simulink model "MIT2"  (R2018a)
settings: Solver=VariableStepAuto  StartTime=0.0  StopTime=200  RelTol=1e-3
settings Model: Creator=boomboom  LastModifiedBy=edward
settings CodeAppCC: StateflowObjectComments=on

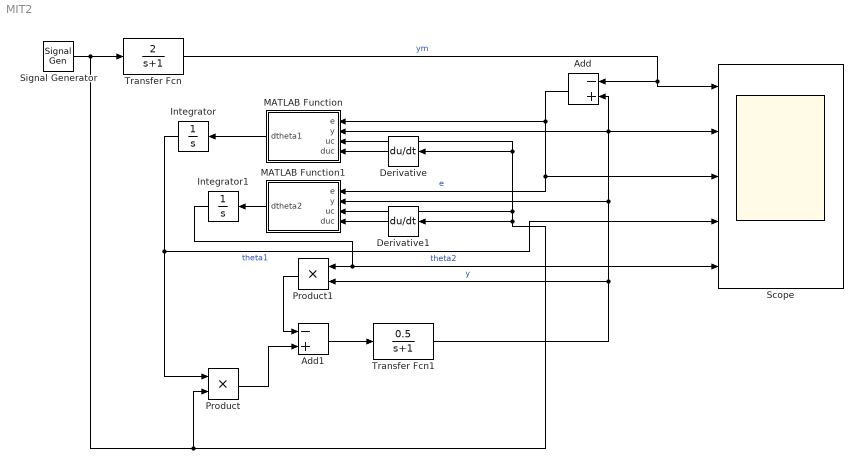
== system MIT2 ==
  Add : Sum  Inputs=-+
  Add1 : Sum  Inputs=-+
  Derivative : Derivative
  Derivative1 : Derivative
  Integrator : Integrator
  Integrator1 : Integrator
  MATLAB Function : MATLAB Function  TreatAsAtomicUnit=on
  MATLAB Function1 : MATLAB Function  TreatAsAtomicUnit=on
  Product : Product
  Product1 : Product
  Scope : Scope  NumInputPorts=5
  Signal Generator : SignalGenerator  Frequency=0.1  Units=rad/sec
  Transfer Fcn : TransferFcn  Numerator=[2]  Denominator=[1 1]
  Transfer Fcn1 : TransferFcn  Numerator=[0.5]  Denominator=[1 1]
  wires:
  Signal Generator/1 -> Product/2, Derivative1/1, Derivative/1, MATLAB Function/3(uc), MATLAB Function1/3(uc), Transfer Fcn/1
  Transfer Fcn/1 -> Add/1, Scope/1  "ym"
  Product/1 -> Add1/2
  Add1/1 -> Transfer Fcn1/1
  Product1/1 -> Add1/1
  Transfer Fcn1/1 -> Product1/2, MATLAB Function1/2(y), MATLAB Function/2(y), Add/2, Scope/2  "y"
  Add/1 -> Scope/3, MATLAB Function1/1(e), MATLAB Function/1(e)  "e"
  Derivative/1 -> MATLAB Function/4(duc)
  Derivative1/1 -> MATLAB Function1/4(duc)
  MATLAB Function/1(dtheta1) -> Integrator/1
  Integrator/1 -> Scope/4, Product/1  "theta1"
  MATLAB Function1/1(dtheta2) -> Integrator1/1
  Integrator1/1 -> Scope/5, Product1/1  "theta2"

== matlab function MIT2/MATLAB Function1 ==
  data: e input; dtheta2 output; y input; uc input; duc input
function dtheta2 = fcn(e,y,uc,duc)
am=2;
bm=2;
a=1;
b=0.5;
gamma=0.2
dtheta2 = -gamma*(am/(duc+am*y))*e

== matlab function MIT2/MATLAB Function ==
  data: e input; dtheta1 output; y input; uc input; duc input
function dtheta1 = fcn(e,y,uc,duc)
am=2;
bm=2;
a=1;
b=0.5;
gamma=0.2
dtheta1 = -gamma*(am/(duc+am*uc))*e
